simulink model "s2_turbine"  (R2019b)
settings: Solver=VariableStepAuto  StartTime=0.0  StopTime=15  RelTol=1e-3
PreLoadFcn:
  | Ts=1;
InitFcn:
  | Ts=1;
libraries: powerlib_meascontrol x1
settings Model: Creator=MAHMUD  LastModifiedBy=MAHMUD

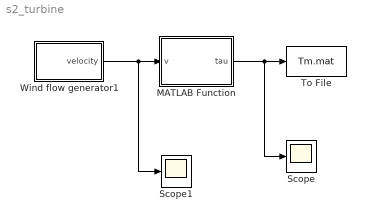
== system s2_turbine ==
  MATLAB Function : MATLAB Function  TreatAsAtomicUnit=on
  Scope : Scope
  Scope1 : Scope
  To File : ToFile  Filename=Tm.mat  SaveFormat=Timeseries
  Wind flow generator1 : Subsystem
  wires:
  MATLAB Function/1(tau) -> Scope/1, To File/1
  Wind flow generator1/1(velocity) -> MATLAB Function/1(v), Scope1/1

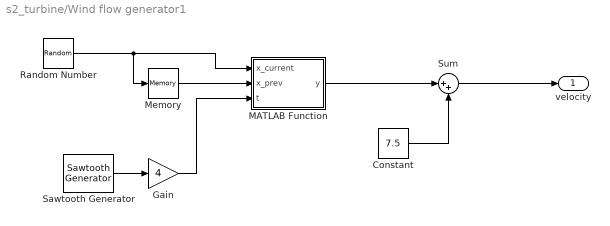
== system s2_turbine/Wind flow generator1 ==
  Constant : Constant  Value=7.5
  Gain : Gain  Gain=4
  MATLAB Function : MATLAB Function  TreatAsAtomicUnit=on
  Memory : Memory  InheritSampleTime=on
  Random Number : RandomNumber  Mean=3  Variance=2  SampleTime=Ts  VectorParams1D=off
  Sawtooth Generator : powerlib_meascontrol/Pulse & Signal Generators/Sawtooth Generator  Freq=1/Ts  Phase=0  Ts=0.001
      settings: SourceProductName=Simscape Electrical
  Sum : Sum  Inputs=|++
  velocity : Outport
  wires:
  Constant/1 -> Sum/2
  Sum/1 -> velocity/1
  Random Number/1 -> MATLAB Function/1(x_current), Memory/1
  Memory/1 -> MATLAB Function/2(x_prev)
  Sawtooth Generator/1 -> Gain/1
  Gain/1 -> MATLAB Function/3(t)
  MATLAB Function/1(y) -> Sum/1

== matlab function s2_turbine/MATLAB Function ==
  data: v input; tau output
function tau = fcn(v)
radius=7;
turbineEfficiency = 0.8;
airDensity=1.2041;
w=8;
c0=0.3906;
c1=0.052;
c2=0.118;
c3=0.16;
c4=0.062;
c5=1.026e-2;
c6=5.65e-4;
powerConst=0.5*pi*(radius^2)*turbineEfficiency*airDensity;

lamda= radius*w/v;
cp=(c1-c2*lamda+c3*lamda^2-c4*lamda^3+c5*lamda^4-c6*lamda^5)*c0;
if(cp<0)
    cp=0;
end
power=powerConst*(v^3)*cp;
tau=power/w;

== matlab function s2_turbine/Wind flow generator1/MATLAB Function ==
  data: x_current input; y output; x_prev input; t input
function y = fcn(x_current,x_prev,t)
y = 2*(((x_current-x_prev)/(1+exp(-t)))+x_prev);
